simulink model "FMU_differential_torque_test"  (R2023b)
settings: Solver=VariableStepAuto  StartTime=0.0  StopTime=100  RelTol=1e-3
settings Model: Creator=denoc  LastModifiedBy=denoc

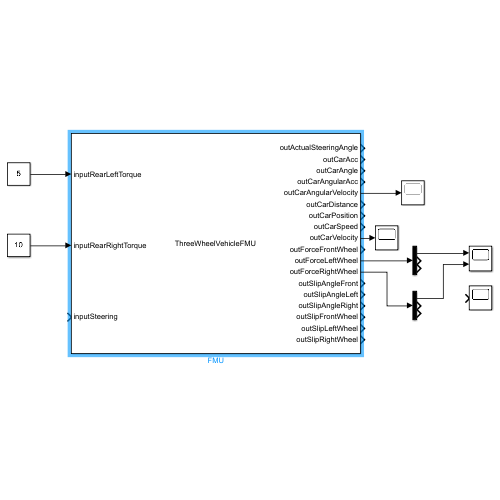
[thumbnail: Simulink's stored preview of the top-level diagram]
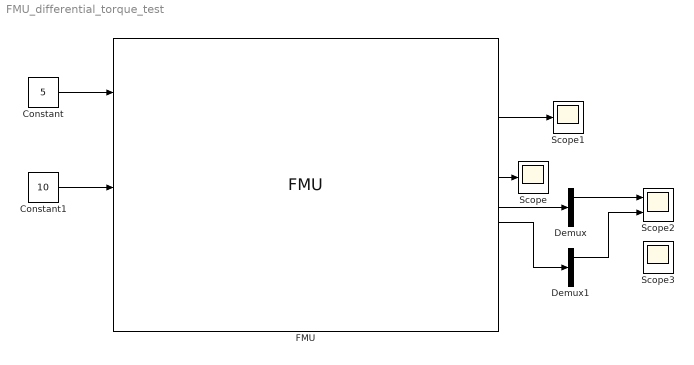
== system FMU_differential_torque_test ==
  Constant : Constant  Value=5
  Constant1 : Constant  Value=10
  Demux : Demux  Outputs=3
  Demux1 : Demux  Outputs=3
  FMU : FMU  FMUName=ThreeWheelVehicleFMU.fmu  FMUMode=ModelExchange  FMUInitializeEnumObject=off  FMUCachedDialogLayout="{\"Geometry\":[154,214,562,418],\"ParameterColumnsWidthConfig\":\"{\\\"columns\\\":[{\\\"name\\\":\\\"Parameter\\\",\\\"width\\\":441},{\\\"name\\\":\\\"Value\\\",\\\"width\\\":332},{\\\"name\\\":\\\"Unit\\\",\\\"width\\\":303},{\\\"name\\\":\\\"Description\\\",\\\"width\\\":463}]}\",\"InputColumnsWidthConfig\":[],\"OutputColumnsWidthConfig\":\"{\\\"columns\\\":[{\\\"name\\\":\\\"Name\\\",\\\"width\\\":216},{\\\"name\\\":\\\"Visibility\\\",\\\"width\\\":79},{\\\"name\\\":\\\"Start\\\",\\\"width\\\":104},{\\\"name\\\":\\\"Unit\\\",\\\"width\\\":101},{\\\"name\\\":\\\"Type Object\\\",\\\"width\\\":157}]}\"}"  airResistanceLongitudinal=struct('r',[0.0,1.0],'rho',1.18)  backLength=0.5  body2=struct('I',1e-08,'m',0.1)  const=struct('k',0.0)  dragCoef=0.5  front=struct('r',[0.0],'width',0.2)  front2=struct('r',[0.001,0.0])  frontLength=1.5  frontTrail=struct('r',[0.0])  frontWheel=struct('diameter',0.1,'r',[0.0,1.0])  g=9.82  gearRatio=7  inertiaBody=350.0  inertiaWheel=0.3  mass=350.0  muA=1.0  muS=0.7  planarWorld=struct('constantGravity',[0.0,0.0],'defaultFrameDiameterFraction',40.0,'defaultN_to_m',1000.0,'defaultNm_to_m',1000.0,'defaultSpecularCoefficient',0.7,'defaultWidthFraction',20.0,'defaultZPosition',0.0,'gravityArrowTail',[0.0,0.0],'nominalLength',1.0)  rear=struct('r',[0.0],'width',0.2)  rearLeft=struct('r',[0,0.0])  rearLeftWheel=struct('diameter',0.1,'r',[0.0,1.0])  rearRight=struct('r',[0,0.0])  rearRightWheel=struct('diameter',0.1,'r',[0.0,1.0])  sAd=0.07000000000000001  sSl=0.2  speedStart=11.11111111111111  steeringControl=struct('i_2',900.0,'p',800.0)  turnRadiusMAX=500.0  vAd=0.1  vSl=0.3  vehicleFrontArea=1.5  vehicleWidth=1.0  wheelRadius=0.28  body_sphere_shapeType=sphere  body2_sphere_shapeType=sphere  front_cylinder_shapeType=cylinder  front2_cylinder_shapeType=cylinder  frontTrail_cylinder_shapeType=cylinder  frontWheel_cylinder_shapeType=cylinder  frontWheel_rim1_shapeType=cylinder  frontWheel_rim2_shapeType=cylinder  planarWorld_label1=x  planarWorld_label2=y  rear_cylinder_shapeType=cylinder  rearLeft_cylinder_shapeType=cylinder  rearLeftWheel_cylinder_shapeType=cylinder  rearLeftWheel_rim1_shapeType=cylinder  rearLeftWheel_rim2_shapeType=cylinder  rearRight_cylinder_shapeType=cylinder  rearRightWheel_cylinder_shapeType=cylinder  rearRightWheel_rim1_shapeType=cylinder  rearRightWheel_rim2_shapeType=cylinder  revolute_cylinder_shapeType=cylinder  mask(ThreeWheelVehicleFMU [Model Exchange, v2.0]){}
      settings: MultithreadedSim=off
      mask Display:
      | disp('ThreeWheelVehicleFMU');
      | port_label('output',1,'outActualSteeringAngle');
      | port_label('output',2,'outCarAcc');
      | port_label('output',3,'outCarAngle');
      | port_label('output',4,'outCarAngularAcc');
      | port_label('output',5,'outCarAngularVelocity');
      | port_label('output',6,'outCarDistance');
      | port_label('output',7,'outCarPosition');
      | port_label('output',8,'outCarSpeed');
      | port_label('output',9,'outCarVelocity');
      | port_label('output',10,'outForceFrontWheel');
      | port_label('output',11,'outForceLeftWheel');
      | port_label('output',12,'outForceRightWheel');
      | port_label('output',13,'outSlipAngleFront');
      | port_label('output',14,'outSlipAngleLeft');
      | port_label('output',15,'outSlipAngleRight');
      | port_label('output',16,'outSlipFrontWheel');
      | port_label('output',17,'outSlipLeftWheel');
      | port_label('output',18,'outSlipRightWheel');
      | port_label('input',1,'inputRearLeftTorque');
      | port_label('input',2,'inputRearRightTorque');
      | port_label('input',3,'inputSteering');
  Scope : Scope
  Scope1 : Scope
  Scope2 : Scope  NumInputPorts=2
  Scope3 : Scope
  wires:
  Constant1/1 -> FMU/2
  Constant/1 -> FMU/1
  FMU/9 -> Scope/1
  FMU/11 -> Demux/1
  FMU/12 -> Demux1/1
  FMU/5 -> Scope1/1
  Demux/1 -> Scope2/1
  Demux1/1 -> Scope2/2
